simulink model "closedloop_model_limit"  (R2024a)
settings: Solver=VariableStepAuto  StartTime=0.0  StopTime=20  RelTol=1e-3
undefined symbols (not defined in the file): Kp, Td, Ti
libraries: cstblocks x2
settings Model: SimulationMode=accelerator  Creator=thoma  LastModifiedBy=thoma

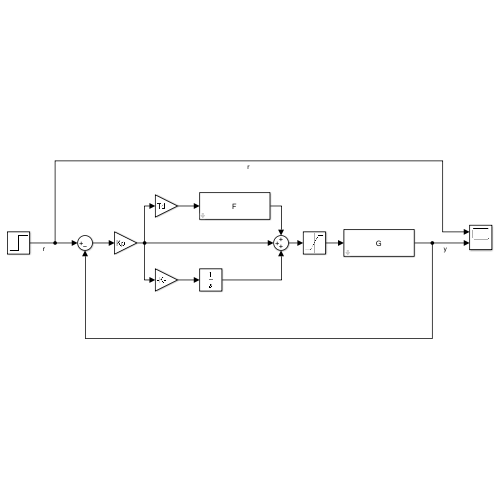
[thumbnail: Simulink's stored preview of the top-level diagram]
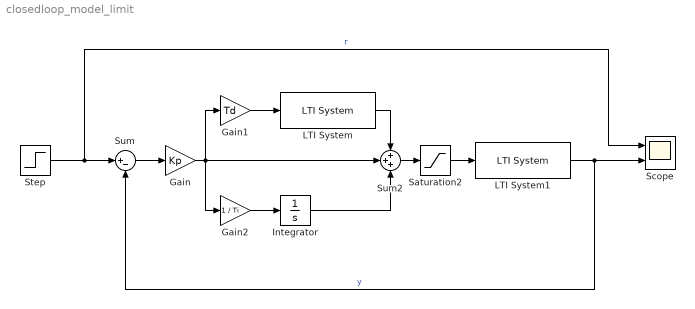
== system closedloop_model_limit ==
  Gain : Gain  Gain=Kp
  Gain1 : Gain  Gain=Td
  Gain2 : Gain  Gain=1 / Ti
  Integrator : Integrator
  LTI System : cstblocks/LTI System  sys=F  IC=[]  PadeOrder=0
  LTI System1 : cstblocks/LTI System  sys=G  IC=[]  PadeOrder=0
  Saturation2 : Saturate  UpperLimit=5  LowerLimit=-5
  Scope : Scope  NumInputPorts=2
  Step : Step  Time=0  SampleTime=0
  Sum : Sum  Inputs=|+-
  Sum2 : Sum  Inputs=+++
  wires:
  Gain/1 -> Gain2/1, Sum2/2, Gain1/1
  Step/1 -> Sum/1, Scope/1  "r"
  Sum/1 -> Gain/1
  Gain1/1 -> LTI System/1
  Gain2/1 -> Integrator/1
  LTI System/1 -> Sum2/1
  LTI System1/1 -> Scope/2, Sum/2  "y"
  Sum2/1 -> Saturation2/1
  Integrator/1 -> Sum2/3
  Saturation2/1 -> LTI System1/1
